simulink model "motor_block_2016b"  (R2016b)
settings: Solver=VariableStepAuto  StartTime=0.0  StopTime=5  RelTol=1e-2
undefined symbols (not defined in the file or in its folder): p, sigbuilder_block, Ts
libraries: nesl_utility x12, fl_lib x11, pe_lib x4, pePwmGenerator x1
settings Model: Creator=HangBiao  LastModifiedBy=HangBiao
settings SolverCC: AlgebraicLoopSolver=LineSearch

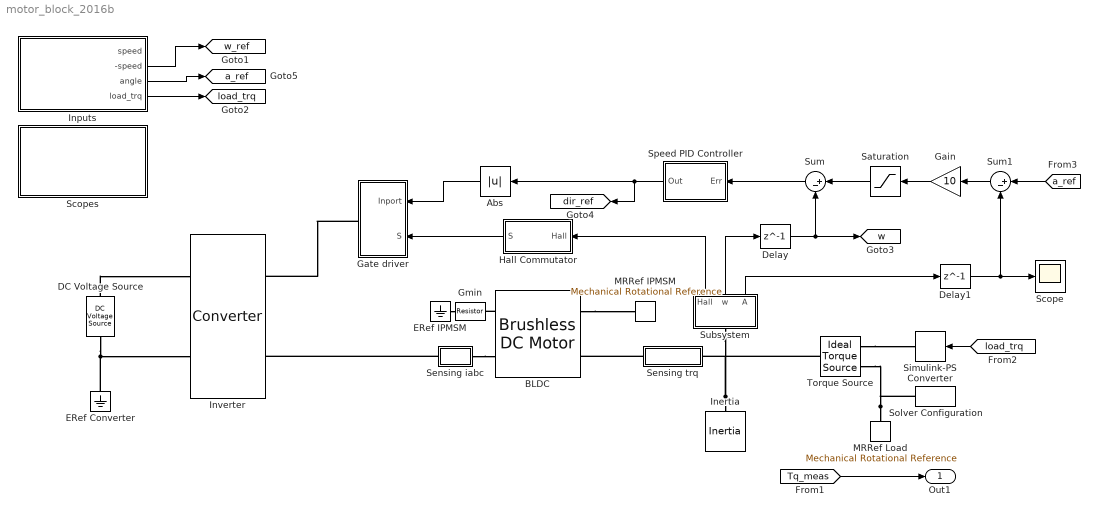
== system motor_block_2016b ==
  Abs : Abs
  BLDC : pe_lib/Machines/Permanent Magnet Rotor/Brushless DC Motor  rotor_param=1  pm_flux_linkage=psim Wb  theta_constant=pi / (2*p) rad  emf_max=9.6 V  DphiDtheta_tab=[0, -.1528, -.1528, .1528, .1528, 0] Wb/rad  back_emf_tab=[0, -9.6, -9.6, 9.6, 9.6, 0] V  rotor_angle_tab=[0, 7.5, 22.5, 37.5, 52.5, 60] deg  w_meas=600 rpm  nPolePairs=p  stator_param=2  Ld=0.00022 H  Lq=0.00022 H  L0=0.00016 H  Ls=Ls H  Lm=0 H  Ms=Ms H  Rs=Rs Ohm  zero_sequence=pe.enum.park.zerosequence.include  J=0.01 kg*m^2  lam=0 N*m/(rad/s)  axes_param=1  i_d_specify=off  i_d_priority=None  i_d=0 A  i_d_nominal_specify=off  i_d_nominal_unit=A  i_d_nominal_value=1  i_q_specify=off  i_q_priority=None  i_q=0 A  i_q_nominal_specify=off  i_q_nominal_unit=A  i_q_nominal_value=1  torque_specify=off  torque_priority=None  torque=0 N*m  torque_nominal_specify=off  torque_nominal_unit=N*m  torque_nominal_value=1  angular_velocity_specify=off  angular_velocity_priority=High  angular_velocity=0 rpm  angular_velocity_nominal_specify=off  angular_velocity_nominal_unit=rpm  angular_velocity_nominal_value=1  angular_position_specify=off  angular_position_priority=High  angular_position=0 deg  angular_position_nominal_specify=off  angular_position_nominal_unit=deg  angular_position_nominal_value=1
  DC Voltage Source : fl_lib/Electrical/Electrical Sources/DC Voltage Source  v0=Vdc V
  Delay : Delay  DelayLength=1  InitialCondition=0
  Delay1 : Delay  DelayLength=1  InitialCondition=0
  ERef Converter : fl_lib/Electrical/Electrical Elements/Electrical Reference
  ERef IPMSM : fl_lib/Electrical/Electrical Elements/Electrical Reference
  Gain : Gain  Gain=10
  Gate driver : Subsystem
  Gmin : fl_lib/Electrical/Electrical Elements/Resistor  R=1e9 Ohm  i_specify=off  i_priority=High  i=0 A  i_nominal_specify=off  i_nominal_unit=A  i_nominal_value=1  v_specify=off  v_priority=High  v=0 V  v_nominal_specify=off  v_nominal_unit=V  v_nominal_value=1
  Hall Commutator : Subsystem
  Inertia : fl_lib/Mechanical/Rotational Elements/Inertia  inertia=Jm kg*m^2  w_specify=on  w_priority=High  w=0 rpm  w_nominal_specify=off  w_nominal_unit=rad/s  w_nominal_value=1  t_specify=off  t_priority=High  t=0 N*m  t_nominal_specify=off  t_nominal_unit=N*m  t_nominal_value=1
  Inputs : Subsystem  Tag=STV Subsys  LoadFcn=sigbuilder_block('load');  StartFcn=sigbuilder_block('start');  StopFcn=sigbuilder_block('stop');  ClipboardFcn=sigbuilder_block('clipboard');  mask(Sigbuilder block){tuvar=[0:10]}
      mask help: Simulink:masks:SigbuilderBlock_MD
      mask init:
      | if ~strcmp(get_param(bdroot(gcbh),'SimulationStatus'),'stopped') tuvar = sigbuilder_block('maskInit'); end
      settings: CopyFcn=sigbuilder_block('copy');  DeleteFcn=sigbuilder_block('delete');  ModelCloseFcn=sigbuilder_block('modelClose');  PreSaveFcn=sigbuilder_block('preSave');  PauseFcn=sigbuilder_block('pause');  ContinueFcn=sigbuilder_block('continue');  NameChangeFcn=sigbuilder_block('namechange');  OpenFcn=sigbuilder_block('open',[249 282 1018 465 ]);  CloseFcn=sigbuilder_block('close');
      mask Display: plot(0, 0, 100, 100,[2, 2, 32, 32, 2], [68, 8, 8, 68, 68],[32, 2], [38, 38], [32, 19, 2],[53, 60, 44], [32, 17, 17, 2],[16, 16, 31, 31]);txt = getActiveGroup(gcbh);text(2, 100, txt,'verticalAlignment', 'top');
  Inverter : pe_lib/Semiconductors/Converter  device_type=3  Vf=0.8 V  Ron=0.001 Ohm  Rds=0.001 Ohm  Goff=1e-5 1/Ohm  Vth=0.5 V  Vgt=1 V  Vgt_off=-1 V  Ih=1 A  diode_param=2  diode_Vf=0.8 V  diode_Ron=0.001 Ohm  diode_Goff=1e-5 1/Ohm  diode_C=50 nF  diode_iRM=-235 A  diode_iF=300 A  diode_idot=-50 A/us  diode_trr_param=1  diode_trr_factor=3  diode_trr=15 us  diode_Qrr=1.5e+3 s*uA  snubber_type=0  Rs=0.1 Ohm  Cs=1e-7 F
  MRRef IPMSM : fl_lib/Mechanical/Rotational Elements/Mechanical Rotational Reference
  MRRef Load : fl_lib/Mechanical/Rotational Elements/Mechanical Rotational Reference
  Saturation : Saturate  UpperLimit=100  LowerLimit=-100
  Scope : Scope
  Scopes : Subsystem
  Sensing trq : Subsystem
      mask Display: disp('trq')
  Sensing iabc : Subsystem
      mask Display: disp('iabc')
  Simulink-PS Converter : nesl_utility/Simulink-PS Converter  PhysicalDomain=network_engine_domain  SubClassName=ps_input  LeftPortType=input  RightPortType=output  PseudoPeriodic=off  Frequencies=[]  NoiseDistribution=none  NoiseParameters=[]  Unit=N*m  AffineConversion=off  FilteringAndDerivatives=zero  SimscapeFilterOrder=1  InputFilterTimeConstant=0.001  UdotUserProvided=1
  Solver Configuration : nesl_utility/Solver Configuration  PhysicalDomain=network_engine_domain  SubClassName=solver  LeftPortType=input  RightPortType=generic  Tones=[]  Harmonics=[]  SimulateNoise=off  Profile=off  UseLocalSampling=off  EnableSwitchedLinearOptims=on  FrequencyDomain=off  UseCCode=off  RelTol=0.001  AbsTol=1e-06  MinStep=1e-09  ToWorkspace=off  RevertToSquareIcSolve=off  NumHomotopyIterations=100  PhasorMode=off  PhasorModeNumHarmonics=1  DoDC=off  ResidualTolerance=1e-9  UseLocalSolver=on  LocalSolverChoice=NE_BACKWARD_EULER_ADVANCER  LocalSolverSampleTime=Ts  DoFixedCost=on  MaxNonlinIter=4  MaxModeIter=2  LinearAlgebra=Sparse  EquationFormulation=NE_TIME_EF  DelaysMemoryBudget=1024  AutomaticFiltering=on  FilteringTimeConstant=0.001
  Speed PID Controller : Subsystem
  Subsystem : Subsystem
  Sum : Sum  Inputs=|+-
  Sum1 : Sum  Inputs=|+-
  Torque Source : fl_lib/Mechanical/Mechanical Sources/Ideal Torque Source
  Out1 : Outport
  tag scope: a_ref=global, dir_ref=global, load_trq=global, w=global, w_ref=global
  wires:
  [load_trq] -> Simulink-PS Converter/1
  Hall Commutator/1(S) -> Gate driver/2(S)
  Subsystem/1(Hall) -> Hall Commutator/1(Hall)
  Delay/1 -> [w], Sum/2
  Gain/1 -> Saturation/1
  Subsystem/2(w) -> Delay/1
  Inputs/4(load_trq) -> [load_trq]
  Sum/1 -> Speed PID Controller/1(Err)
  Speed PID Controller/1(Out) -> [dir_ref], Abs/1
  Inputs/2(-speed) -> [w_ref]
  Abs/1 -> Gate driver/1(Inport)
  Inputs/3(angle) -> [a_ref]
  [a_ref] -> Sum1/1
  Sum1/1 -> Gain/1
  Subsystem/3(A) -> Delay1/1
  Delay1/1 -> Scope/1, Sum1/2
  Saturation/1 -> Sum/1
  [Tq_meas] -> Out1/1
  connections:
  Inertia/LConn1 -- Torque Source/LConn1 -- Subsystem/LConn1 -- Sensing trq/RConn1
  MRRef Load/LConn1 -- Torque Source/RConn2 -- Solver Configuration/RConn1
  ERef Converter/LConn1 -- DC Voltage Source/RConn1 -- Inverter/RConn2
  Torque Source/RConn1 -- Simulink-PS Converter/RConn1
  ERef IPMSM/LConn1 -- Gmin/LConn1
  Sensing iabc/RConn1 -- BLDC/LConn1
  Gate driver/RConn1 -- Inverter/LConn1
  BLDC/RConn2 -- MRRef IPMSM/LConn1
  Sensing trq/LConn1 -- BLDC/RConn1
  DC Voltage Source/LConn1 -- Inverter/RConn1
  BLDC/LConn2 -- Gmin/RConn1
  Sensing iabc/LConn1 -- Inverter/LConn2

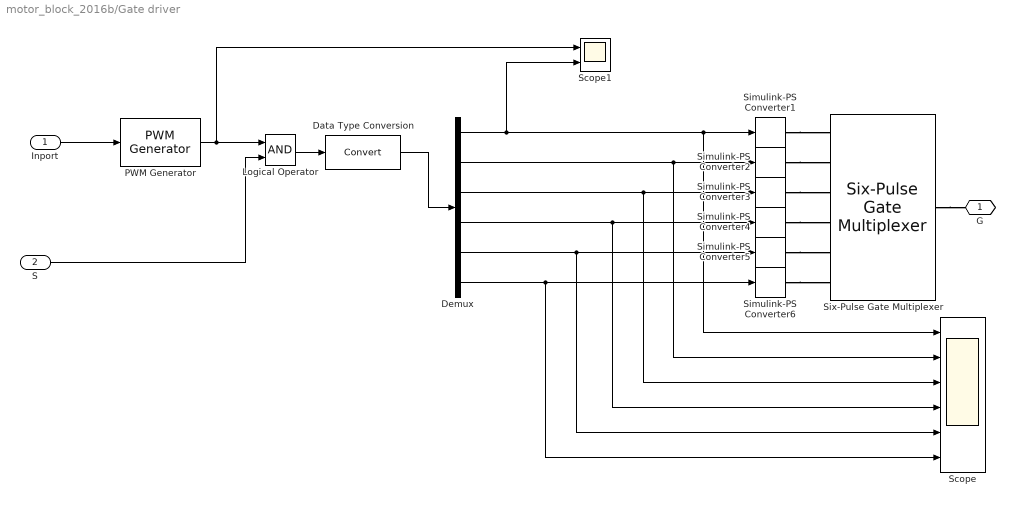
== system motor_block_2016b/Gate driver ==
  Inport : Inport
  S : Inport  Port=2
  Data Type Conversion : DataTypeConversion
  Demux : Demux  Outputs=6
  Logical Operator : Logic  AllPortsSameDT=off  OutDataTypeStr=boolean
  PWM Generator : pePwmGenerator/PWM Generator  CarrCount=Up  Tper=Tsc  Ts=Ts
  Scope : Scope  NumInputPorts=6
  Scope1 : Scope  NumInputPorts=2
  Simulink-PS Converter{1..6} (6 alike) : nesl_utility/Simulink-PS Converter  PhysicalDomain=network_engine_domain  SubClassName=ps_input  LeftPortType=input  RightPortType=output  PseudoPeriodic=off  Frequencies=[]  NoiseDistribution=none  NoiseParameters=[]  Unit=1  AffineConversion=off  FilteringAndDerivatives=zero  SimscapeFilterOrder=1  InputFilterTimeConstant=0.001  UdotUserProvided=1
  Six-Pulse Gate Multiplexer : pe_lib/Semiconductors/Six-Pulse Gate Multiplexer  R=0 Ohm
  G : PMIOPort  Side=Right
  wires:
  Demux/4 -> Scope/4, Simulink-PS Converter4/1
  Demux/2 -> Scope/2, Simulink-PS Converter2/1
  Demux/3 -> Scope/3, Simulink-PS Converter3/1
  Demux/5 -> Scope/5, Simulink-PS Converter5/1
  Demux/6 -> Scope/6, Simulink-PS Converter6/1
  Inport/1 -> PWM Generator/1
  PWM Generator/1 -> Scope1/1, Logical Operator/1
  Logical Operator/1 -> Data Type Conversion/1
  Demux/1 -> Scope1/2, Scope/1, Simulink-PS Converter1/1
  S/1 -> Logical Operator/2
  Data Type Conversion/1 -> Demux/1
  connections:
  Six-Pulse Gate Multiplexer/RConn1 -- G/RConn1
  Simulink-PS Converter1/RConn1 -- Six-Pulse Gate Multiplexer/LConn1
  Simulink-PS Converter3/RConn1 -- Six-Pulse Gate Multiplexer/LConn3
  Simulink-PS Converter5/RConn1 -- Six-Pulse Gate Multiplexer/LConn5
  Simulink-PS Converter6/RConn1 -- Six-Pulse Gate Multiplexer/LConn6
  Simulink-PS Converter4/RConn1 -- Six-Pulse Gate Multiplexer/LConn4
  Simulink-PS Converter2/RConn1 -- Six-Pulse Gate Multiplexer/LConn2

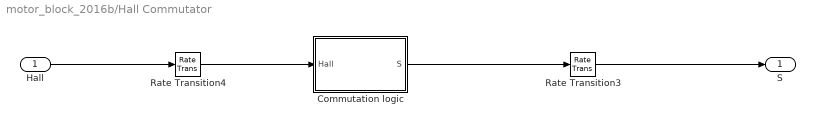
== system motor_block_2016b/Hall Commutator ==
  Hall : Inport
  Commutation logic : Subsystem
  Rate Transition3 : RateTransition  OutPortSampleTime=Ts
  Rate Transition4 : RateTransition  OutPortSampleTime=Tsc
  S : Outport
  wires:
  Rate Transition3/1 -> S/1
  Hall/1 -> Rate Transition4/1
  Commutation logic/1(S) -> Rate Transition3/1
  Rate Transition4/1 -> Commutation logic/1(Hall)

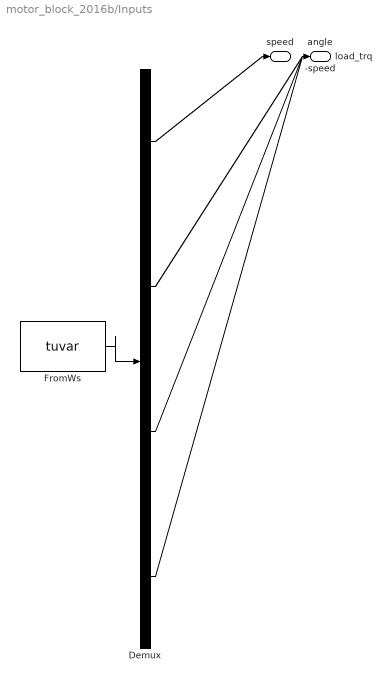
== system motor_block_2016b/Inputs ==
  Demux : Demux  Tag=STV Demux
  FromWs : FromWorkspace  Tag=STV FromWs  VariableName=tuvar  SampleTime=0
      SigBuilderData=|
      | common.afterFinalStr = 'Extrapolate'
      | common.sampleTime = 0
      | dataSet.timeRange = [0 1]
      | dataSet.name = 'Input'
      | sbobj.Groups.Name = 'Input'
      | sbobj.Groups.Signals(1).Name = 'speed'
      | sbobj.Groups.Signals(1).XData = [0 1]
      | sbobj.Groups.Signals(1).YData = [50 50]
      | sbobj.Groups.Signals(2).Name = '-speed'
      | sbobj.Groups.Signals(2).XData = [0 1]
      | sbobj.Groups.Signals(2).YData = [-50 -50]
      | sbobj.Groups.Signals(3).Name = 'angle'
      | sbobj.Groups.Signals(3).XData = [0 1]
      | sbobj.Groups.Signals(3).YData = [100 100]
      | sbobj.Groups.Signals(4).Name = 'load_trq'
      | sbobj.Groups.Signals(4).XData = [0 1]
      | sbobj.Groups.Signals(4).YData = [-1.7 -1.7]
      | sbobj.Groups.TimeRange = [0 1]
  speed : Outport  Tag=STV Outport
  -speed : Outport  Tag=STV Outport  Port=2
  angle : Outport  Tag=STV Outport  Port=3
  load_trq : Outport  Tag=STV Outport  Port=4
  wires:
  FromWs/1 -> Demux/1
  Demux/1 -> speed/1
  Demux/2 -> -speed/1
  Demux/3 -> angle/1
  Demux/4 -> load_trq/1

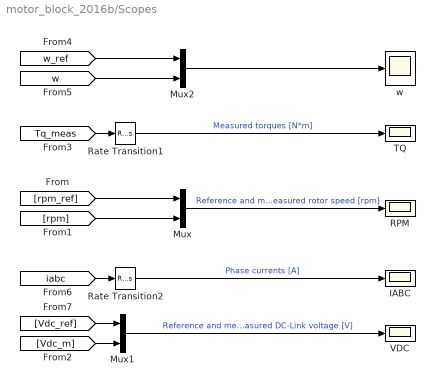
== system motor_block_2016b/Scopes ==
  IABC : Scope
  Mux : Mux  Inputs=2
  Mux1 : Mux  Inputs=2
  Mux2 : Mux  Inputs=2
  RPM : Scope
  Rate Transition1 : RateTransition
  Rate Transition2 : RateTransition  OutPortSampleTime=1e-4
  TQ : Scope
  VDC : Scope
  w : Scope
  wires:
  [rpm] -> Mux/2
  Mux1/1 -> VDC/1  "Reference and measured DC-Link voltage [V]"
  [Vdc_ref] -> Mux1/1
  Rate Transition2/1 -> IABC/1  "Phase currents [A]"
  [rpm_ref] -> Mux/1
  [iabc] -> Rate Transition2/1
  [Tq_meas] -> Rate Transition1/1
  Rate Transition1/1 -> TQ/1  "Measured torques [N*m]"
  Mux/1 -> RPM/1  "Reference and measured rotor speed [rpm]"
  [Vdc_m] -> Mux1/2
  [w_ref] -> Mux2/1
  [w] -> Mux2/2
  Mux2/1 -> w/1

== system motor_block_2016b/Sensing trq ==
  PS-Simulink Converter3 : nesl_utility/PS-Simulink Converter  PhysicalDomain=network_engine_domain  SubClassName=ps_output  LeftPortType=input  RightPortType=output  PseudoPeriodic=off  Frequencies=[]  Unit=N*m  AffineConversion=off
  Torque Sensor : fl_lib/Mechanical/Mechanical Sensors/Ideal Torque Sensor
  R : PMIOPort  Side=Left
  C : PMIOPort  Port=2  Side=Right
  tag scope: Tq_meas=global
  wires:
  PS-Simulink Converter3/1 -> [Tq_meas]
  connections:
  Torque Sensor/RConn1 -- C/RConn1
  Torque Sensor/RConn2 -- PS-Simulink Converter3/LConn1
  Torque Sensor/LConn1 -- R/RConn1

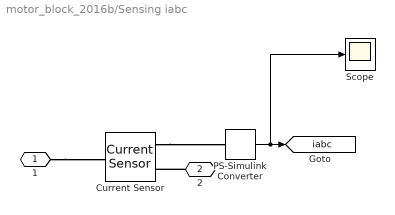
== system motor_block_2016b/Sensing iabc ==
  Current Sensor : pe_lib/Sensors/Current Sensor
  PS-Simulink Converter : nesl_utility/PS-Simulink Converter  PhysicalDomain=network_engine_domain  SubClassName=ps_output  LeftPortType=input  RightPortType=output  PseudoPeriodic=off  Frequencies=[]  Unit=A  AffineConversion=off
  Scope : Scope
  1 : PMIOPort  Side=Left
  2 : PMIOPort  Port=2  Side=Right
  tag scope: iabc=global
  wires:
  PS-Simulink Converter/1 -> Scope/1, [iabc]
  connections:
  1/RConn1 -- Current Sensor/LConn1
  2/RConn1 -- Current Sensor/RConn2
  Current Sensor/RConn1 -- PS-Simulink Converter/LConn1

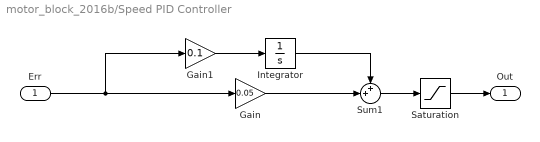
== system motor_block_2016b/Speed PID Controller ==
  Err : Inport
  Gain : Gain  Gain=0.05
  Gain1 : Gain  Gain=0.1
  Integrator : Integrator
  Saturation : Saturate  UpperLimit=1  LowerLimit=-1
  Sum1 : Sum  Inputs=++|
  Out : Outport
  wires:
  Saturation/1 -> Out/1
  Integrator/1 -> Sum1/1
  Sum1/1 -> Saturation/1
  Gain/1 -> Sum1/2
  Gain1/1 -> Integrator/1
  Err/1 -> Gain1/1, Gain/1

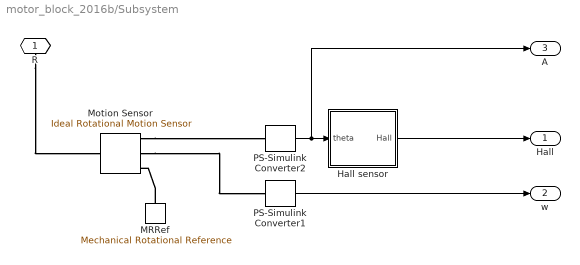
== system motor_block_2016b/Subsystem ==
  Hall sensor : Subsystem
  MRRef : fl_lib/Mechanical/Rotational Elements/Mechanical Rotational Reference
  Motion Sensor : fl_lib/Mechanical/Mechanical Sensors/Ideal Rotational Motion Sensor  offset=0 deg
  PS-Simulink Converter1 : nesl_utility/PS-Simulink Converter  PhysicalDomain=network_engine_domain  SubClassName=ps_output  LeftPortType=input  RightPortType=output  PseudoPeriodic=off  Frequencies=[]  Unit=rad/s  AffineConversion=off
  PS-Simulink Converter2 : nesl_utility/PS-Simulink Converter  PhysicalDomain=network_engine_domain  SubClassName=ps_output  LeftPortType=input  RightPortType=output  PseudoPeriodic=off  Frequencies=[]  Unit=rad  AffineConversion=off
  R : PMIOPort  Side=Left
  Hall : Outport
  w : Outport  Port=2
  A : Outport  Port=3
  wires:
  PS-Simulink Converter1/1 -> w/1
  Hall sensor/1(Hall) -> Hall/1
  PS-Simulink Converter2/1 -> A/1, Hall sensor/1(theta)
  connections:
  R/RConn1 -- Motion Sensor/LConn1
  MRRef/LConn1 -- Motion Sensor/RConn1
  Motion Sensor/RConn3 -- PS-Simulink Converter2/LConn1
  Motion Sensor/RConn2 -- PS-Simulink Converter1/LConn1

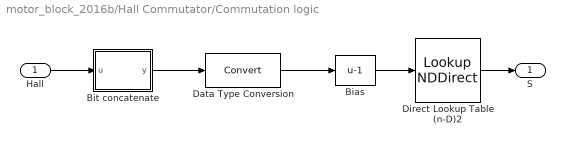
== system motor_block_2016b/Hall Commutator/Commutation logic ==
  Hall : Inport
  Bias : Bias  Bias=-1
  Bit concatenate : Subsystem
  Data Type Conversion : DataTypeConversion
  Direct Lookup Table (n-D)2 : LookupNDDirect  InputsSelectThisObjectFromTable=Column  Table=[0 0 0 1 1 0;0 1 1 0 0 0;0 1 0 0 0 1;1 0 0 0 1 0;1 0 1 0 0 0;0 0 0 1 0 1]
  S : Outport
  wires:
  Hall/1 -> Bit concatenate/1(u)
  Bit concatenate/1(y) -> Data Type Conversion/1
  Direct Lookup Table (n-D)2/1 -> S/1
  Data Type Conversion/1 -> Bias/1
  Bias/1 -> Direct Lookup Table (n-D)2/1

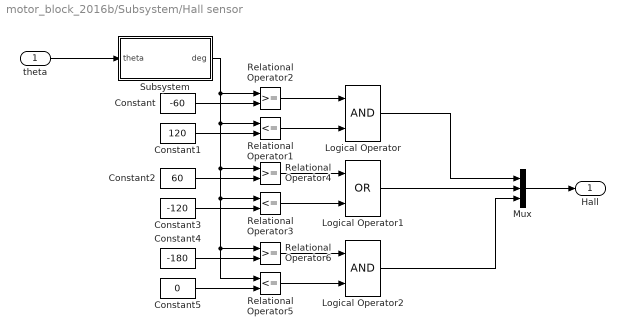
== system motor_block_2016b/Subsystem/Hall sensor ==
  theta : Inport
  Constant : Constant  Value=-60
  Constant1 : Constant  Value=120
  Constant2 : Constant  Value=60
  Constant3 : Constant  Value=-120
  Constant4 : Constant  Value=-180
  Constant5 : Constant  Value=0
  Logical Operator : Logic  AllPortsSameDT=off  OutDataTypeStr=boolean
  Logical Operator1 : Logic  Operator=OR  AllPortsSameDT=off  OutDataTypeStr=boolean
  Logical Operator2 : Logic  AllPortsSameDT=off  OutDataTypeStr=boolean
  Mux : Mux  Inputs=3
  Relational Operator1 : RelationalOperator  Operator=<=  RndMeth=Nearest  InputSameDT=on
  Relational Operator2 : RelationalOperator  RndMeth=Nearest  InputSameDT=on
  Relational Operator3 : RelationalOperator  Operator=<=  RndMeth=Nearest  InputSameDT=on
  Relational Operator4 : RelationalOperator  RndMeth=Nearest  InputSameDT=on
  Relational Operator5 : RelationalOperator  Operator=<=  RndMeth=Nearest  InputSameDT=on
  Relational Operator6 : RelationalOperator  RndMeth=Nearest  InputSameDT=on
  Subsystem : Subsystem
  Hall : Outport
  wires:
  Constant3/1 -> Relational Operator3/2
  Logical Operator2/1 -> Mux/3
  Logical Operator1/1 -> Mux/2
  Logical Operator/1 -> Mux/1
  Relational Operator5/1 -> Logical Operator2/2
  Relational Operator6/1 -> Logical Operator2/1
  Constant4/1 -> Relational Operator6/2
  Constant5/1 -> Relational Operator5/2
  Relational Operator3/1 -> Logical Operator1/2
  Mux/1 -> Hall/1
  Relational Operator2/1 -> Logical Operator/1
  Relational Operator1/1 -> Logical Operator/2
  Subsystem/1(deg) -> Relational Operator4/1, Relational Operator3/1, Relational Operator5/1, Relational Operator6/1, Relational Operator1/1, Relational Operator2/1
  Constant/1 -> Relational Operator2/2
  Relational Operator4/1 -> Logical Operator1/1
  Constant1/1 -> Relational Operator1/2
  Constant2/1 -> Relational Operator4/2
  theta/1 -> Subsystem/1(theta)

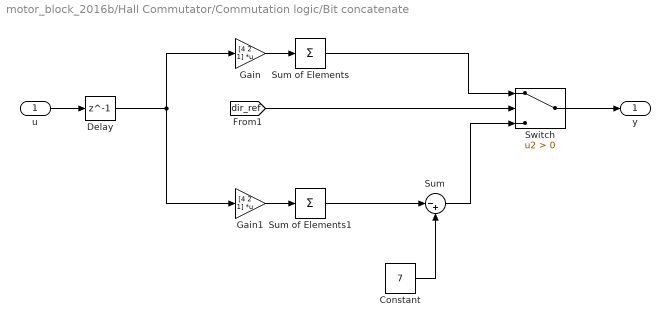
== system motor_block_2016b/Hall Commutator/Commutation logic/Bit concatenate ==
  u : Inport
  Constant : Constant  Value=7
  Delay : Delay  DelayLength=1  InitialCondition=0
  Gain : Gain  Gain=[4 2 1]  Multiplication=Matrix(K*u)
  Gain1 : Gain  Gain=[4 2 1]  Multiplication=Matrix(K*u)
  Sum : Sum  Inputs=|-+
  Sum of Elements : Sum  Inputs=+
  Sum of Elements1 : Sum  Inputs=+
  Switch : Switch  Criteria=u2 > Threshold
  y : Outport
  wires:
  Gain/1 -> Sum of Elements/1
  [dir_ref] -> Switch/2
  Switch/1 -> y/1
  Sum of Elements/1 -> Switch/1
  u/1 -> Delay/1
  Gain1/1 -> Sum of Elements1/1
  Sum of Elements1/1 -> Sum/1
  Sum/1 -> Switch/3
  Constant/1 -> Sum/2
  Delay/1 -> Gain/1, Gain1/1

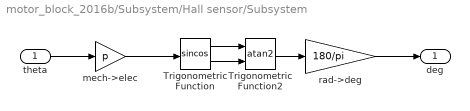
== system motor_block_2016b/Subsystem/Hall sensor/Subsystem ==
  theta : Inport
  Trigonometric Function : Trigonometry  Operator=sincos
  Trigonometric Function2 : Trigonometry  Operator=atan2
  mech->elec : Gain  Gain=p
  rad->deg : Gain  Gain=180/pi  SaturateOnIntegerOverflow=on  OutDataTypeStr=Inherit: Same as input  ParamDataTypeStr=Inherit: Same as input
  deg : Outport
  wires:
  Trigonometric Function2/1 -> rad->deg/1
  Trigonometric Function/1 -> Trigonometric Function2/1
  theta/1 -> mech->elec/1
  rad->deg/1 -> deg/1
  Trigonometric Function/2 -> Trigonometric Function2/2
  mech->elec/1 -> Trigonometric Function/1
